simulink model "gm_IPCore_3Level_PWM"  (R2025b)
settings: Solver=VariableStepAuto  StartTime=0.0  StopTime=0.0004  RelTol=1e-3
undefined symbols (not defined in the file or in its folder): f_Carrier, f_FPGA_clk, T_FPGA_clk
libraries: hdlmdlgenlib x4, hdlsllib x3
settings Model: Creator=info  LastModifiedBy=info
settings OptimizationCC: BlockReduction=off  ConditionallyExecuteInputs=off  DefaultParameterBehavior=Inlined
settings DebuggingCC: AlgebraicLoopMsg=error  InheritedTsInSrcMsg=none  SingleTaskRateTransMsg=error
settings HardwareCC: ProdBitPerPointer=32.0  ProdBitPerSizeT=32.0  ProdBitPerPtrDiffT=32.0  ProdLargestAtomicFloat=None  ProdIntDivRoundTo=Undefined  ProdEndianess=Unspecified  ProdWordSize=32.0  ProdHWDeviceType=ASIC/FPGA->ASIC/FPGA  TargetBitPerPointer=64.0  TargetBitPerSizeT=64.0  TargetBitPerPtrDiffT=64.0  TargetLongLongMode=on  TargetIntDivRoundTo=Zero  TargetEndianess=LittleEndian  TargetWordSize=64.0  TargetHWDeviceType=Custom Processor->MATLAB Host Computer  ProdEqTarget=off

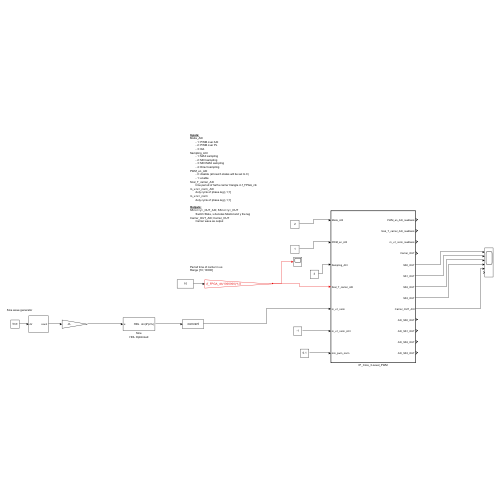
[thumbnail: Simulink's stored preview of the top-level diagram]
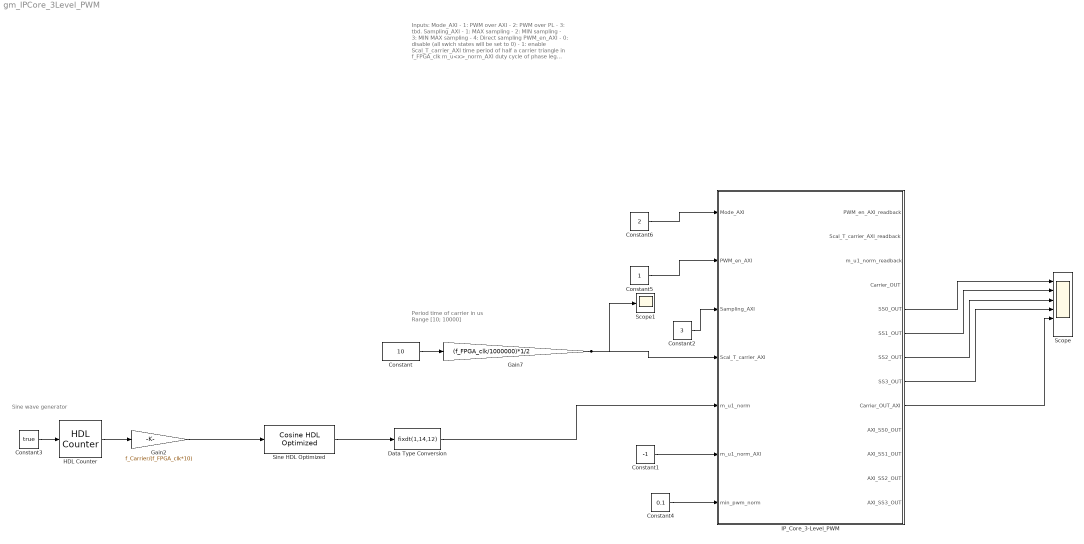
== system gm_IPCore_3Level_PWM ==
  note: Period time of carrier in us
      | Range [10; 10000]
  note: Inputs:
      | Mode_AXI
      | - 1: PWM over AXI
      | - 2: PWM over PL
      | - 3: tbd.
      | Sampling_AXI
      | - 1: MAX sampling
      | - 2: MIN sampling
      | - 3: MIN MAX sampling
      | - 4: Direct sampling
      | PWM_en_AXI
      | - 0: disable (all swich states will be set to 0)
      | - 1: enable
      | Scal_T_carrier_AXI
      | time period of half a carrier triangle in f_FPGA_clk
      | m_u<x>_norm_AXI
      | duty cycle of phase leg [-1;1]
      | m_u<x>_norm
      | duty cycle of phase leg [-1;1]
      |
      | Outputs:
      | SS<x><y>_OUT_AXI; SS<x><y>_OUT
      | Switch State, x denotes Mosfet and y the leg
      | Carrier_OUT_AXI; Carrier_OUT
      | Carrier wave as output
  note: Sine wave generator
  Constant : Constant  Value=10  SampleTime=T_FPGA_clk
  Constant1 : Constant  Value=-1  OutDataTypeStr=fixdt(1,14,12)  SampleTime=T_FPGA_clk
  Constant2 : Constant  Value=3  OutDataTypeStr=uint8  SampleTime=T_FPGA_clk
  Constant3 : Constant  Value=true  OutDataTypeStr=boolean  SampleTime=T_FPGA_clk
  Constant4 : Constant  Value=0.1  OutDataTypeStr=fixdt(0,13,12)
  Constant5 : Constant  OutDataTypeStr=boolean  SampleTime=T_FPGA_clk
  Constant6 : Constant  Value=2  OutDataTypeStr=uint8  SampleTime=T_FPGA_clk
  Data Type Conversion : DataTypeConversion  OutDataTypeStr=fixdt(1,14,12)  SaturateOnIntegerOverflow=off  RndMeth=Floor
  Gain2 : Gain  Gain=f_Carrier/(f_FPGA_clk*10)
  Gain7 : Gain  Gain=(f_FPGA_clk/1000000)*1/2  OutDataTypeStr=fixdt(0,25,0)
  HDL Counter : hdlsllib/Sources/HDL Counter  CountType=Free running  CountInit=0  CountStep=1  CountMax=25  CountFromType=Initial value  CountFrom=0  CountResetPort=off  CountLoadPort=off  CountEnbPort=off  CountDirPort=on  CountHitOutputPort=off  CountDataType=Unsigned  CountWordLen=20  CountFracLen=0  CountSampTime=1
  IP_Core_3-Level_PWM : Subsystem  TreatAsAtomicUnit=on
  Scope : Scope  NumInputPorts=6
      settings: ActiveDisplayYMinimum=-0.12499999999999997  ActiveDisplayYMaximum=1.125  DataLoggingVariableName=ScopeData2  DataLoggingSaveFormat=Array
  Scope1 : Scope
      settings: ActiveDisplayYMinimum=-2.0551334999999995E+6  ActiveDisplayYMaximum=1.85012015E+7  DataLoggingSaveFormat=Array
  Sine HDL Optimized : hdlsllib/Lookup Tables/Cosine HDL Optimized  OutputFormula=sin(2*pi*u)  NumDataPoints=64  TableDataTypeStr=fixdt(0,16,15)  SimulateLUTROMDelay=off
      settings: LibrarySourceBlock=|
      | hdlsllib/Lookup
      | Tables/Sine
      | HDL Optimized
  wires:
  Constant4/1 -> IP_Core_3-Level_PWM/7(min_pwm_norm)
  Constant1/1 -> IP_Core_3-Level_PWM/6(m_u1_norm_AXI)
  Constant6/1 -> IP_Core_3-Level_PWM/1(Mode_AXI)
  IP_Core_3-Level_PWM/8(SS3_OUT) -> Scope/4
  IP_Core_3-Level_PWM/7(SS2_OUT) -> Scope/3
  IP_Core_3-Level_PWM/6(SS1_OUT) -> Scope/2
  Constant2/1 -> IP_Core_3-Level_PWM/3(Sampling_AXI)
  IP_Core_3-Level_PWM/9(Carrier_OUT_AXI) -> Scope/5
  Data Type Conversion/1 -> IP_Core_3-Level_PWM/5(m_u1_norm)
  IP_Core_3-Level_PWM/5(SS0_OUT) -> Scope/1
  Constant5/1 -> IP_Core_3-Level_PWM/2(PWM_en_AXI)
  Sine HDL Optimized/1 -> Data Type Conversion/1
  Constant3/1 -> HDL Counter/1
  HDL Counter/1 -> Gain2/1
  Gain2/1 -> Sine HDL Optimized/1
  Gain7/1 -> Scope1/1, IP_Core_3-Level_PWM/4(Scal_T_carrier_AXI)
  Constant/1 -> Gain7/1

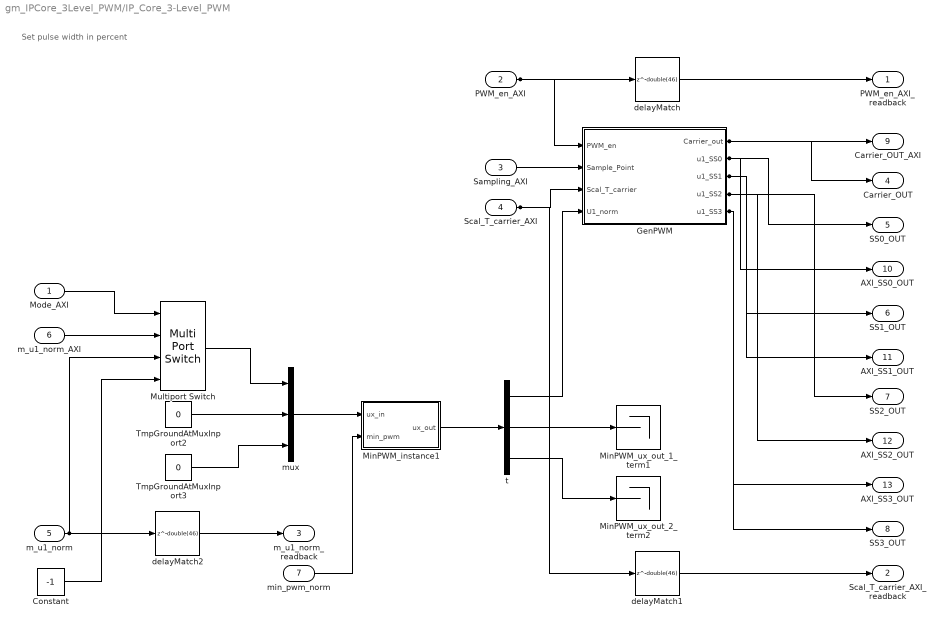
== system gm_IPCore_3Level_PWM/IP_Core_3-Level_PWM ==
  note: Set pulse width in percent
  Mode_AXI : Inport  OutDataTypeStr=uint8  PortDimensions=1  SampleTime=1e-08
  PWM_en_AXI : Inport  Port=2  OutDataTypeStr=boolean  PortDimensions=1  SampleTime=1e-08
  Sampling_AXI : Inport  Port=3  OutDataTypeStr=uint8  PortDimensions=1  SampleTime=1e-08
  Scal_T_carrier_AXI : Inport  Port=4  OutDataTypeStr=fixdt(0, 25, 0)  PortDimensions=1  SampleTime=1e-08
  m_u1_norm : Inport  Port=5  OutDataTypeStr=fixdt(1, 14, 12)  PortDimensions=1  SampleTime=1e-08
  m_u1_norm_AXI : Inport  Port=6  OutDataTypeStr=fixdt(1, 14, 12)  PortDimensions=1  SampleTime=1e-08
  min_pwm_norm : Inport  Port=7  OutDataTypeStr=fixdt(0, 13, 12)  PortDimensions=1  SampleTime=1e-08
  Constant : Constant  Value=-1  OutDataTypeStr=fixdt(1, 14, 12)  SampleTime=1e-08
  GenPWM : Subsystem
  MinPWM_instance1 : Subsystem
  MinPWM_ux_out_1_term1 : Terminator
  MinPWM_ux_out_2_term2 : Terminator
  Multiport Switch : MultiPortSwitch  DiagnosticForDefault=None  OutDataTypeStr=fixdt(1, 14, 12)  SampleTime=1e-08  SaturateOnIntegerOverflow=off  InputSameDT=off
  TmpGroundAtMuxInport2 : Constant  Value=0  VectorParams1D=off  OutDataTypeStr=fixdt(1, 14, 12)  SampleTime=1e-08
  TmpGroundAtMuxInport3 : Constant  Value=0  VectorParams1D=off  OutDataTypeStr=fixdt(1, 14, 12)  SampleTime=1e-08
  delayMatch : Delay  DelayLength=double(46)  InitialCondition=0  SampleTime=1e-08
  delayMatch1 : Delay  DelayLength=double(46)  InitialCondition=0  SampleTime=1e-08
  delayMatch2 : Delay  DelayLength=double(46)  InitialCondition=0  SampleTime=1e-08
  mux : Mux  Inputs=3
  t : Demux  Outputs=3
  PWM_en_AXI_readback : Outport  SampleTime=1e-08  VectorParamsAs1DForOutWhenUnconnected=off
  Scal_T_carrier_AXI_readback : Outport  Port=2  SampleTime=1e-08
  m_u1_norm_readback : Outport  Port=3  SampleTime=1e-08
  Carrier_OUT : Outport  Port=4  SampleTime=1e-08
  SS0_OUT : Outport  Port=5  SampleTime=1e-08  VectorParamsAs1DForOutWhenUnconnected=off
  SS1_OUT : Outport  Port=6  SampleTime=1e-08  VectorParamsAs1DForOutWhenUnconnected=off
  SS2_OUT : Outport  Port=7  SampleTime=1e-08  VectorParamsAs1DForOutWhenUnconnected=off
  SS3_OUT : Outport  Port=8  SampleTime=1e-08  VectorParamsAs1DForOutWhenUnconnected=off
  Carrier_OUT_AXI : Outport  Port=9  SampleTime=1e-08
  AXI_SS0_OUT : Outport  Port=10  SampleTime=1e-08
  AXI_SS1_OUT : Outport  Port=11  SampleTime=1e-08
  AXI_SS2_OUT : Outport  Port=12  SampleTime=1e-08
  AXI_SS3_OUT : Outport  Port=13  SampleTime=1e-08
  wires:
  TmpGroundAtMuxInport2/1 -> mux/2
  Mode_AXI/1 -> Multiport Switch/1
  delayMatch2/1 -> m_u1_norm_readback/1
  m_u1_norm_AXI/1 -> Multiport Switch/2
  TmpGroundAtMuxInport3/1 -> mux/3
  t/3 -> MinPWM_ux_out_2_term2/1
  m_u1_norm/1 -> delayMatch2/1, Multiport Switch/3
  Constant/1 -> Multiport Switch/4
  Multiport Switch/1 -> mux/1
  delayMatch/1 -> PWM_en_AXI_readback/1
  mux/1 -> MinPWM_instance1/1(ux_in)
  GenPWM/4(u1_SS2) -> SS2_OUT/1, AXI_SS2_OUT/1
  min_pwm_norm/1 -> MinPWM_instance1/2(min_pwm)
  MinPWM_instance1/1(ux_out) -> t/1
  PWM_en_AXI/1 -> delayMatch/1, GenPWM/1(PWM_en)
  Sampling_AXI/1 -> GenPWM/2(Sample_Point)
  Scal_T_carrier_AXI/1 -> delayMatch1/1, GenPWM/3(Scal_T_carrier)
  t/1 -> GenPWM/4(U1_norm)
  t/2 -> MinPWM_ux_out_1_term1/1
  GenPWM/1(Carrier_out) -> Carrier_OUT/1, Carrier_OUT_AXI/1
  GenPWM/2(u1_SS0) -> SS0_OUT/1, AXI_SS0_OUT/1
  GenPWM/3(u1_SS1) -> SS1_OUT/1, AXI_SS1_OUT/1
  GenPWM/5(u1_SS3) -> AXI_SS3_OUT/1, SS3_OUT/1
  delayMatch1/1 -> Scal_T_carrier_AXI_readback/1

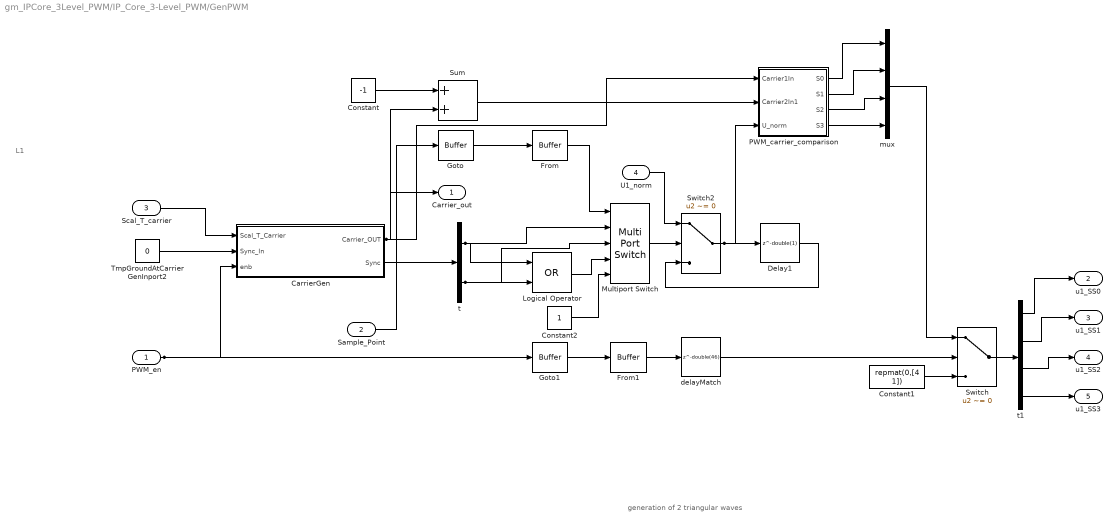
== system gm_IPCore_3Level_PWM/IP_Core_3-Level_PWM/GenPWM ==
  note: generation of 2 triangular waves
  note: L1
  PWM_en : Inport  OutDataTypeStr=boolean  PortDimensions=1  SampleTime=1e-08
  Sample_Point : Inport  Port=2  OutDataTypeStr=uint8  PortDimensions=1  SampleTime=1e-08
  Scal_T_carrier : Inport  Port=3  OutDataTypeStr=fixdt(0, 25, 0)  PortDimensions=1  SampleTime=1e-08
  U1_norm : Inport  Port=4  OutDataTypeStr=fixdt(1, 28, 25)  PortDimensions=1  SampleTime=1e-08
  CarrierGen : Subsystem
  Constant : Constant  Value=-1  OutDataTypeStr=fixdt(1, 14, 12)  SampleTime=1e-08
  Constant1 : Constant  Value="repmat(0,[4  1])"  OutDataTypeStr=fixdt(0, 1, 0)  SampleTime=1e-08
  Constant2 : Constant  OutDataTypeStr=fixdt(0, 1, 0)  SampleTime=1e-08
  Delay1 : Delay  DelayLength=double(1)  InitialCondition=0  SampleTime=1e-08
  From : hdlmdlgenlib/Buffer
  From1 : hdlmdlgenlib/Buffer
  Goto : hdlmdlgenlib/Buffer
  Goto1 : hdlmdlgenlib/Buffer
  Logical Operator : Logic  Operator=OR  AllPortsSameDT=off  OutDataTypeStr=fixdt(0, 1, 0)  SampleTime=1e-08
  Multiport Switch : MultiPortSwitch  Inputs=4  DiagnosticForDefault=None  SampleTime=1e-08  SaturateOnIntegerOverflow=off  InputSameDT=off
  PWM_carrier_comparison : Subsystem
  Sum : Sum  OutDataTypeStr=fixdt(1, 19, 16)  AccumDataTypeStr=fixdt(1, 19, 16)  SampleTime=1e-08
  Switch : Switch  Criteria=u2 ~= 0  Threshold="fi(0,0,1,0,\"hex\",\"0\")"  OutDataTypeStr=boolean  SampleTime=1e-08  SaturateOnIntegerOverflow=off  InputSameDT=off
  Switch2 : Switch  Criteria=u2 ~= 0  Threshold="fi(0,0,1,0,\"hex\",\"0\")"  OutDataTypeStr=fixdt(1, 28, 25)  SampleTime=1e-08  SaturateOnIntegerOverflow=off  InputSameDT=off
  TmpGroundAtCarrierGenInport2 : Constant  Value=0  VectorParams1D=off  OutDataTypeStr=boolean  SampleTime=1e-08
  delayMatch : Delay  DelayLength=double(46)  InitialCondition=0  SampleTime=1e-08
  mux : Mux
  t : Demux  Outputs=2
  t1 : Demux
  Carrier_out : Outport  SampleTime=1e-08
  u1_SS0 : Outport  Port=2  SampleTime=1e-08
  u1_SS1 : Outport  Port=3  SampleTime=1e-08
  u1_SS2 : Outport  Port=4  SampleTime=1e-08
  u1_SS3 : Outport  Port=5  SampleTime=1e-08
  wires:
  CarrierGen/1(Carrier_OUT) -> PWM_carrier_comparison/1(Carrier1In), Sum/2, Carrier_out/1
  t1/4 -> u1_SS3/1
  t1/3 -> u1_SS2/1
  t1/2 -> u1_SS1/1
  t1/1 -> u1_SS0/1
  Scal_T_carrier/1 -> CarrierGen/1(Scal_T_Carrier)
  Goto/1 -> From/1
  Sample_Point/1 -> Goto/1
  TmpGroundAtCarrierGenInport2/1 -> CarrierGen/2(Sync_In)
  Constant/1 -> Sum/1
  From1/1 -> delayMatch/1
  PWM_en/1 -> Goto1/1, CarrierGen/3(enb)
  CarrierGen/2(Sync) -> t/1
  Sum/1 -> PWM_carrier_comparison/2(Carrier2In1)
  t/2 -> Multiport Switch/3, Logical Operator/2
  t/1 -> Multiport Switch/2, Logical Operator/1
  Constant1/1 -> Switch/3
  From/1 -> Multiport Switch/1
  Logical Operator/1 -> Multiport Switch/4
  Constant2/1 -> Multiport Switch/5
  Goto1/1 -> From1/1
  U1_norm/1 -> Switch2/1
  Multiport Switch/1 -> Switch2/2
  Switch2/1 -> Delay1/1, PWM_carrier_comparison/3(U_norm)
  delayMatch/1 -> Switch/2
  PWM_carrier_comparison/2(S1) -> mux/2
  PWM_carrier_comparison/1(S0) -> mux/1
  Delay1/1 -> Switch2/3
  PWM_carrier_comparison/3(S2) -> mux/3
  PWM_carrier_comparison/4(S3) -> mux/4
  mux/1 -> Switch/1
  Switch/1 -> t1/1

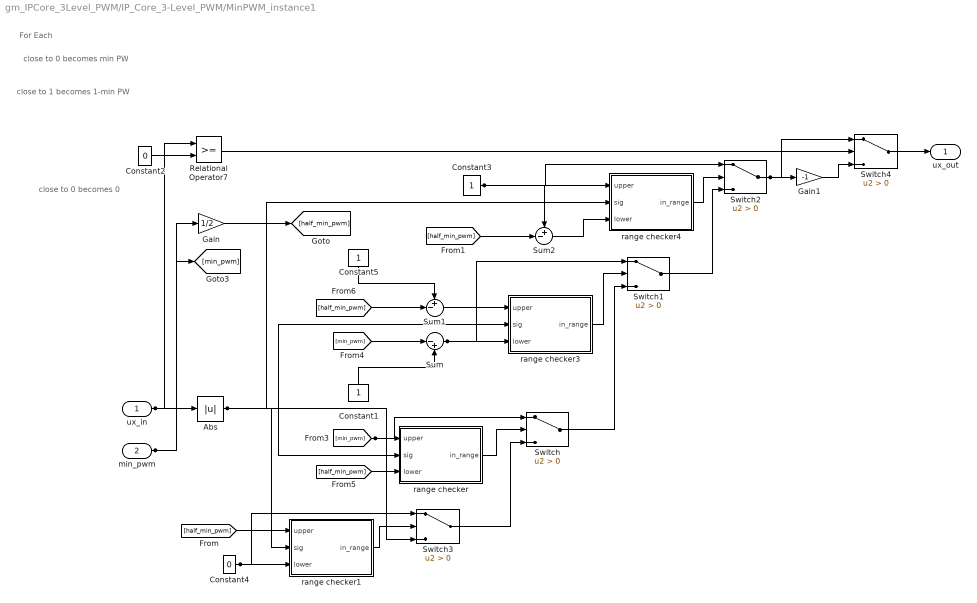
== system gm_IPCore_3Level_PWM/IP_Core_3-Level_PWM/MinPWM_instance1 ==
  note: For Each
  note: close to 0 becomes 0
  note: close to 1 becomes 1-min PW
  note: close to 0 becomes min PW
  ux_in : Inport  OutDataTypeStr=fixdt(1, 14, 12)  PortDimensions=[3 1]  SampleTime=1e-08
  min_pwm : Inport  Port=2  OutDataTypeStr=fixdt(0, 13, 12)  PortDimensions=1  SampleTime=1e-08
  Abs : Abs  OutDataTypeStr=fixdt(1, 14, 12)  SaturateOnIntegerOverflow=off
  Constant1 : Constant  OutDataTypeStr=fixdt(0,13,12)  SampleTime=T_FPGA_clk
  Constant2 : Constant  Value=0  OutDataTypeStr=fixdt(0,13,12)  SampleTime=T_FPGA_clk
  Constant3 : Constant  OutDataTypeStr=fixdt(0,13,12)  SampleTime=T_FPGA_clk
  Constant4 : Constant  Value=0  OutDataTypeStr=fixdt(0,13,12)  SampleTime=T_FPGA_clk
  Constant5 : Constant  OutDataTypeStr=fixdt(0,13,12)  SampleTime=T_FPGA_clk
  Gain : Gain  Gain=1/2  OutDataTypeStr=fixdt(0, 26, 25)
  Gain1 : Gain  Gain=-1  OutDataTypeStr=fixdt(1, 28, 25)
  Relational Operator7 : RelationalOperator  OutDataTypeStr=boolean  RndMeth=Simplest  InputSameDT=off
  Sum : Sum  Inputs=|-+  OutDataTypeStr=fixdt(1, 14, 12)
  Sum1 : Sum  Inputs=+-|  OutDataTypeStr=fixdt(1, 27, 25)
  Sum2 : Sum  Inputs=+-|  OutDataTypeStr=fixdt(1, 27, 25)
  Switch : Switch  Criteria=u2 > Threshold  OutDataTypeStr=fixdt(1,14,12)  SaturateOnIntegerOverflow=off  InputSameDT=off
  Switch1 : Switch  Criteria=u2 > Threshold  OutDataTypeStr=fixdt(1, 14, 12)  SaturateOnIntegerOverflow=off  InputSameDT=off
  Switch2 : Switch  Criteria=u2 > Threshold  OutDataTypeStr=fixdt(1, 14, 12)  SaturateOnIntegerOverflow=off  InputSameDT=off
  Switch3 : Switch  Criteria=u2 > Threshold  OutDataTypeStr=fixdt(1, 14, 12)  SaturateOnIntegerOverflow=off  InputSameDT=off
  Switch4 : Switch  Criteria=u2 > Threshold  OutDataTypeStr=fixdt(1, 28, 25)  SaturateOnIntegerOverflow=off  InputSameDT=off
  range checker : Subsystem
  range checker1 : Subsystem
  range checker3 : Subsystem
  range checker4 : Subsystem
  ux_out : Outport  SampleTime=1e-08
  wires:
  Constant3/1 -> Sum2/1, Switch2/1, range checker4/1(upper)
  Constant2/1 -> Relational Operator7/2
  ux_in/1 -> Abs/1, Relational Operator7/1
  Relational Operator7/1 -> Switch4/2
  range checker/1(in_range) -> Switch/2
  min_pwm/1 -> Gain/1, [min_pwm]
  Abs/1 -> Switch3/3, range checker/2(sig), range checker3/2(sig), range checker4/2(sig), range checker1/2(sig)
  Gain/1 -> [half_min_pwm]
  [half_min_pwm] -> Sum2/2
  [half_min_pwm] -> range checker1/1(upper)
  Constant5/1 -> Sum1/1
  Constant4/1 -> Switch3/1, range checker1/3(lower)
  [half_min_pwm] -> range checker/3(lower)
  [half_min_pwm] -> Sum1/2
  [min_pwm] -> Switch/1, range checker/1(upper)
  [min_pwm] -> Sum/1
  Constant1/1 -> Sum/2
  range checker1/1(in_range) -> Switch3/2
  Sum1/1 -> range checker3/1(upper)
  Sum/1 -> Switch1/1, range checker3/3(lower)
  Switch3/1 -> Switch/3
  Sum2/1 -> range checker4/3(lower)
  range checker3/1(in_range) -> Switch1/2
  Switch/1 -> Switch1/3
  range checker4/1(in_range) -> Switch2/2
  Switch1/1 -> Switch2/3
  Switch2/1 -> Switch4/1, Gain1/1
  Gain1/1 -> Switch4/3
  Switch4/1 -> ux_out/1

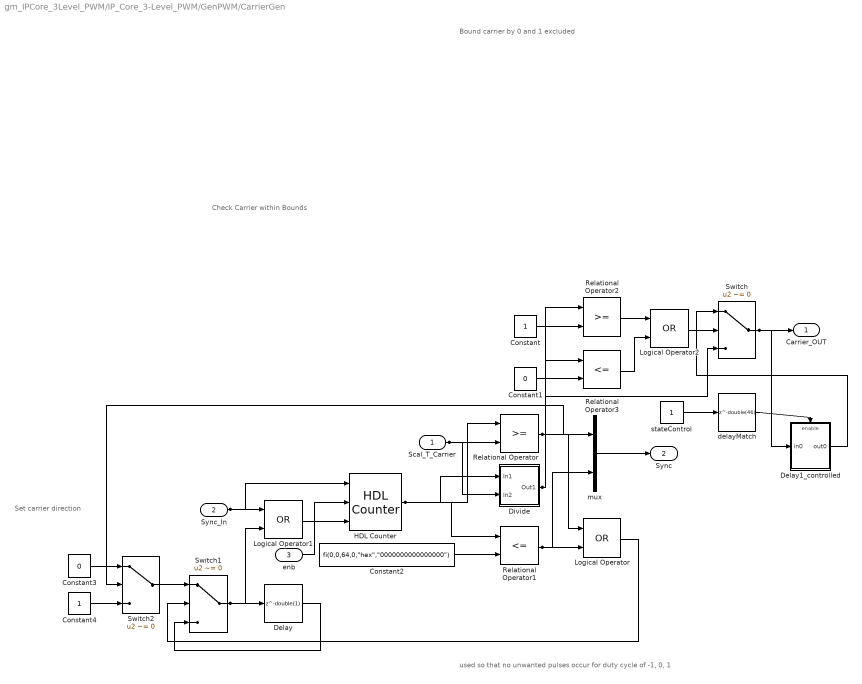
== system gm_IPCore_3Level_PWM/IP_Core_3-Level_PWM/GenPWM/CarrierGen ==
  note: Check Carrier within Bounds
  note: Set carrier direction
  note: Bound carrier by 0 and 1 excluded
  note: used so that no unwanted pulses occur for duty cycle of -1, 0, 1
  Scal_T_Carrier : Inport  OutDataTypeStr=fixdt(0, 25, 0)  PortDimensions=1  SampleTime=1e-08
  Sync_In : Inport  Port=2  OutDataTypeStr=boolean  PortDimensions=1  SampleTime=1e-08
  enb : Inport  Port=3  OutDataTypeStr=boolean  PortDimensions=1  SampleTime=1e-08
  Constant : Constant  OutDataTypeStr=fixdt(1, 18, 16)  SampleTime=1e-08
  Constant1 : Constant  Value=0  OutDataTypeStr=fixdt(1, 18, 16)  SampleTime=1e-08
  Constant2 : Constant  Value="fi(0,0,64,0,\"hex\",\"0000000000000000\")"  OutDataTypeStr=fixdt(0, 64, 0)  SampleTime=1e-08
  Constant3 : Constant  Value=0  OutDataTypeStr=boolean  SampleTime=1e-08
  Constant4 : Constant  OutDataTypeStr=boolean  SampleTime=1e-08
  Delay : Delay  DelayLength=double(1)  InitialCondition=0  SampleTime=1e-08
  Delay1_controlled : Subsystem
  Divide : Subsystem
  HDL Counter : hdlsllib/Sources/HDL Counter  CountType=Free running  CountInit=0  CountStep=1  CountMax=25  CountFromType=Initial value  CountFrom=0  CountResetPort=on  CountLoadPort=off  CountEnbPort=on  CountDirPort=on  CountHitOutputPort=off  CountDataType=Unsigned  CountWordLen=20  CountFracLen=0  CountSampTime=1
  Logical Operator : Logic  Operator=OR  AllPortsSameDT=off  OutDataTypeStr=boolean  SampleTime=1e-08
  Logical Operator1 : Logic  Operator=OR  AllPortsSameDT=off  OutDataTypeStr=boolean  SampleTime=1e-08
  Logical Operator2 : Logic  Operator=OR  AllPortsSameDT=off  OutDataTypeStr=boolean  SampleTime=1e-08
  Relational Operator : RelationalOperator  OutDataTypeStr=boolean  SampleTime=1e-08  InputSameDT=off
  Relational Operator1 : RelationalOperator  Operator=<=  OutDataTypeStr=boolean  SampleTime=1e-08  InputSameDT=off
  Relational Operator2 : RelationalOperator  OutDataTypeStr=boolean  SampleTime=1e-08  InputSameDT=off
  Relational Operator3 : RelationalOperator  Operator=<=  OutDataTypeStr=boolean  SampleTime=1e-08  InputSameDT=off
  Switch : Switch  Criteria=u2 ~= 0  Threshold="fi(0,0,1,0,\"hex\",\"0\")"  OutDataTypeStr=fixdt(1, 18, 16)  SampleTime=1e-08  SaturateOnIntegerOverflow=off  InputSameDT=off
  Switch1 : Switch  Criteria=u2 ~= 0  Threshold="fi(0,0,1,0,\"hex\",\"0\")"  OutDataTypeStr=boolean  SampleTime=1e-08  SaturateOnIntegerOverflow=off  InputSameDT=off
  Switch2 : Switch  Criteria=u2 ~= 0  Threshold="fi(0,0,1,0,\"hex\",\"0\")"  OutDataTypeStr=boolean  SampleTime=1e-08  SaturateOnIntegerOverflow=off  InputSameDT=off
  delayMatch : Delay  DelayLength=double(46)  InitialCondition=0  SampleTime=1e-08
  mux : Mux  Inputs=2
  stateControl : Constant  OutDataTypeStr=boolean  SampleTime=1e-08
  Carrier_OUT : Outport  SampleTime=1e-08
  Sync : Outport  Port=2  SampleTime=1e-08
  wires:
  Logical Operator1/1 -> HDL Counter/3
  Constant3/1 -> Switch2/1
  Constant4/1 -> Switch2/3
  Switch2/1 -> Switch1/1
  Sync_In/1 -> HDL Counter/1, Logical Operator1/1
  Switch1/1 -> Delay/1, Logical Operator1/2
  enb/1 -> HDL Counter/2
  Delay/1 -> Switch1/3
  Scal_T_Carrier/1 -> Divide/2(In2), Relational Operator/2
  HDL Counter/1 -> Relational Operator1/1, Relational Operator/1, Divide/1(In1)
  Constant1/1 -> Relational Operator3/2
  Constant2/1 -> Relational Operator1/2
  Constant/1 -> Relational Operator2/2
  Relational Operator/1 -> Logical Operator/1, mux/1, Switch2/2
  Divide/1(Out1) -> Switch/3, Relational Operator3/1, Relational Operator2/1
  Relational Operator1/1 -> mux/2, Logical Operator/2
  mux/1 -> Sync/1
  Relational Operator2/1 -> Logical Operator2/1
  Relational Operator3/1 -> Logical Operator2/2
  Logical Operator/1 -> Switch1/2
  Logical Operator2/1 -> Switch/2
  stateControl/1 -> delayMatch/1
  Switch/1 -> Delay1_controlled/1(in0), Carrier_OUT/1
  delayMatch/1 -> Delay1_controlled/Enable
  Delay1_controlled/1(out0) -> Switch/1

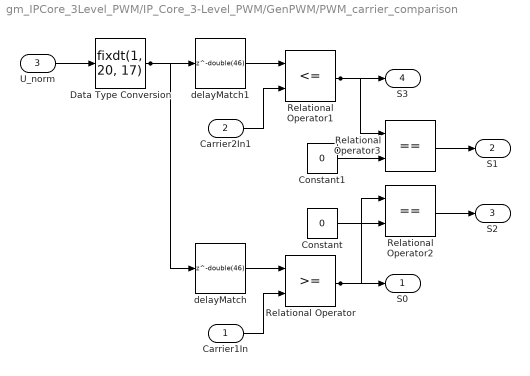
== system gm_IPCore_3Level_PWM/IP_Core_3-Level_PWM/GenPWM/PWM_carrier_comparison ==
  Carrier1In : Inport  OutDataTypeStr=fixdt(1, 18, 16)  PortDimensions=1  SampleTime=1e-08
  Carrier2In1 : Inport  Port=2  OutDataTypeStr=fixdt(1, 19, 16)  PortDimensions=1  SampleTime=1e-08
  U_norm : Inport  Port=3  OutDataTypeStr=fixdt(1, 28, 25)  PortDimensions=1  SampleTime=1e-08
  Constant : Constant  Value=0  OutDataTypeStr=fixdt(0, 1, 0)  SampleTime=1e-08
  Constant1 : Constant  Value=0  OutDataTypeStr=fixdt(0, 1, 0)  SampleTime=1e-08
  Data Type Conversion : DataTypeConversion  OutDataTypeStr=fixdt(1, 20, 17)  RndMeth=Nearest  SampleTime=1e-08  SaturateOnIntegerOverflow=off
  Relational Operator : RelationalOperator  OutDataTypeStr=fixdt(0, 1, 0)  SampleTime=1e-08  InputSameDT=off
  Relational Operator1 : RelationalOperator  Operator=<=  OutDataTypeStr=fixdt(0, 1, 0)  SampleTime=1e-08  InputSameDT=off
  Relational Operator2 : RelationalOperator  Operator===  OutDataTypeStr=fixdt(0, 1, 0)  SampleTime=1e-08  InputSameDT=off
  Relational Operator3 : RelationalOperator  Operator===  OutDataTypeStr=fixdt(0, 1, 0)  SampleTime=1e-08  InputSameDT=off
  delayMatch : Delay  DelayLength=double(46)  InitialCondition=0  SampleTime=1e-08
  delayMatch1 : Delay  DelayLength=double(46)  InitialCondition=0  SampleTime=1e-08
  S0 : Outport  SampleTime=1e-08
  S1 : Outport  Port=2  SampleTime=1e-08
  S2 : Outport  Port=3  SampleTime=1e-08
  S3 : Outport  Port=4  SampleTime=1e-08
  wires:
  U_norm/1 -> Data Type Conversion/1
  Relational Operator1/1 -> Relational Operator3/1, S3/1
  Carrier2In1/1 -> Relational Operator1/2
  Data Type Conversion/1 -> delayMatch1/1, delayMatch/1
  delayMatch1/1 -> Relational Operator1/1
  delayMatch/1 -> Relational Operator/1
  Carrier1In/1 -> Relational Operator/2
  Constant1/1 -> Relational Operator3/2
  Constant/1 -> Relational Operator2/2
  Relational Operator/1 -> Relational Operator2/1, S0/1
  Relational Operator3/1 -> S1/1
  Relational Operator2/1 -> S2/1

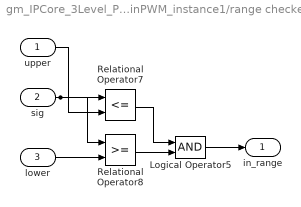
== system gm_IPCore_3Level_PWM/IP_Core_3-Level_PWM/MinPWM_instance1/range checker ==
  upper : Inport  OutDataTypeStr=fixdt(0, 13, 12)  PortDimensions=1  SampleTime=1e-08
  sig : Inport  Port=2  OutDataTypeStr=fixdt(1, 14, 12)  PortDimensions=[3 1]  SampleTime=1e-08
  lower : Inport  Port=3  OutDataTypeStr=fixdt(0, 26, 25)  PortDimensions=1  SampleTime=1e-08
  Logical Operator5 : Logic  AllPortsSameDT=off  OutDataTypeStr=boolean
  Relational Operator7 : RelationalOperator  Operator=<=  OutDataTypeStr=boolean  RndMeth=Simplest  InputSameDT=off
  Relational Operator8 : RelationalOperator  OutDataTypeStr=boolean  RndMeth=Simplest  InputSameDT=off
  in_range : Outport  SampleTime=1e-08
  wires:
  Relational Operator8/1 -> Logical Operator5/2
  upper/1 -> Relational Operator7/2
  Relational Operator7/1 -> Logical Operator5/1
  sig/1 -> Relational Operator7/1, Relational Operator8/1
  Logical Operator5/1 -> in_range/1
  lower/1 -> Relational Operator8/2

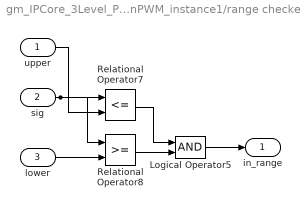
== system gm_IPCore_3Level_PWM/IP_Core_3-Level_PWM/MinPWM_instance1/range checker1 ==
  upper : Inport  OutDataTypeStr=fixdt(0, 26, 25)  PortDimensions=1  SampleTime=1e-08
  sig : Inport  Port=2  OutDataTypeStr=fixdt(1, 14, 12)  PortDimensions=[3 1]  SampleTime=1e-08
  lower : Inport  Port=3  OutDataTypeStr=fixdt(0, 13, 12)  PortDimensions=1  SampleTime=1e-08
  Logical Operator5 : Logic  AllPortsSameDT=off  OutDataTypeStr=boolean
  Relational Operator7 : RelationalOperator  Operator=<=  OutDataTypeStr=boolean  RndMeth=Simplest  InputSameDT=off
  Relational Operator8 : RelationalOperator  OutDataTypeStr=boolean  RndMeth=Simplest  InputSameDT=off
  in_range : Outport  SampleTime=1e-08
  wires:
  Relational Operator8/1 -> Logical Operator5/2
  upper/1 -> Relational Operator7/2
  Relational Operator7/1 -> Logical Operator5/1
  sig/1 -> Relational Operator7/1, Relational Operator8/1
  Logical Operator5/1 -> in_range/1
  lower/1 -> Relational Operator8/2

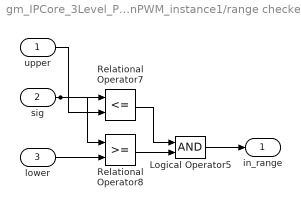
== system gm_IPCore_3Level_PWM/IP_Core_3-Level_PWM/MinPWM_instance1/range checker3 ==
  upper : Inport  OutDataTypeStr=fixdt(1, 27, 25)  PortDimensions=1  SampleTime=1e-08
  sig : Inport  Port=2  OutDataTypeStr=fixdt(1, 14, 12)  PortDimensions=[3 1]  SampleTime=1e-08
  lower : Inport  Port=3  OutDataTypeStr=fixdt(1, 14, 12)  PortDimensions=1  SampleTime=1e-08
  Logical Operator5 : Logic  AllPortsSameDT=off  OutDataTypeStr=boolean
  Relational Operator7 : RelationalOperator  Operator=<=  OutDataTypeStr=boolean  RndMeth=Simplest  InputSameDT=off
  Relational Operator8 : RelationalOperator  OutDataTypeStr=boolean  RndMeth=Simplest  InputSameDT=off
  in_range : Outport  SampleTime=1e-08
  wires:
  upper/1 -> Relational Operator7/2
  sig/1 -> Relational Operator7/1, Relational Operator8/1
  Logical Operator5/1 -> in_range/1
  lower/1 -> Relational Operator8/2
  Relational Operator7/1 -> Logical Operator5/1
  Relational Operator8/1 -> Logical Operator5/2

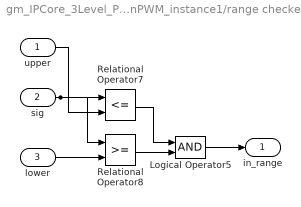
== system gm_IPCore_3Level_PWM/IP_Core_3-Level_PWM/MinPWM_instance1/range checker4 ==
  upper : Inport  OutDataTypeStr=fixdt(0, 13, 12)  PortDimensions=1  SampleTime=1e-08
  sig : Inport  Port=2  OutDataTypeStr=fixdt(1, 14, 12)  PortDimensions=[3 1]  SampleTime=1e-08
  lower : Inport  Port=3  OutDataTypeStr=fixdt(1, 27, 25)  PortDimensions=1  SampleTime=1e-08
  Logical Operator5 : Logic  AllPortsSameDT=off  OutDataTypeStr=boolean
  Relational Operator7 : RelationalOperator  Operator=<=  OutDataTypeStr=boolean  RndMeth=Simplest  InputSameDT=off
  Relational Operator8 : RelationalOperator  OutDataTypeStr=boolean  RndMeth=Simplest  InputSameDT=off
  in_range : Outport  SampleTime=1e-08
  wires:
  upper/1 -> Relational Operator7/2
  sig/1 -> Relational Operator7/1, Relational Operator8/1
  lower/1 -> Relational Operator8/2
  Relational Operator7/1 -> Logical Operator5/1
  Logical Operator5/1 -> in_range/1
  Relational Operator8/1 -> Logical Operator5/2

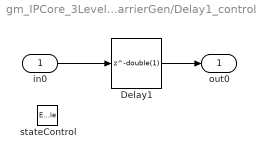
== system gm_IPCore_3Level_PWM/IP_Core_3-Level_PWM/GenPWM/CarrierGen/Delay1_controlled ==
  in0 : Inport  OutDataTypeStr=fixdt(1,18,16,'DataTypeOverride', 'Off')  SampleTime=1e-08
  stateControl : EnablePort  OutDataTypeStr=boolean
  Delay1 : Delay  DelayLength=double(1)  InitialCondition=0  SampleTime=1e-08
  out0 : Outport  OutDataTypeStr=fixdt(1,18,16,'DataTypeOverride', 'Off')  SampleTime=1e-08
  wires:
  in0/1 -> Delay1/1
  Delay1/1 -> out0/1

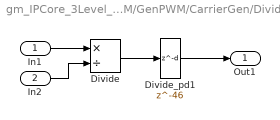
== system gm_IPCore_3Level_PWM/IP_Core_3-Level_PWM/GenPWM/CarrierGen/Divide ==
  In1 : Inport
  In2 : Inport  Port=2
  Divide : Product  Inputs=*/  OutDataTypeStr=fixdt(1,18,16)  RndMeth=Zero  SaturateOnIntegerOverflow=on
  Divide_pd1 : Delay  DelayLength=46
  Out1 : Outport
  wires:
  In1/1 -> Divide/1
  Divide_pd1/1 -> Out1/1
  In2/1 -> Divide/2
  Divide/1 -> Divide_pd1/1
